simulink model "Tarea_4"  (R2013a)
settings: Solver=ode23s  StartTime=0.0  StopTime=10.0  RelTol=1e-3
libraries: simulink x6
settings Model: Creator=Miguel  LastModifiedBy=Miguel
settings DataIOCC: LimitDataPoints=off  MaxDataPoints=10000

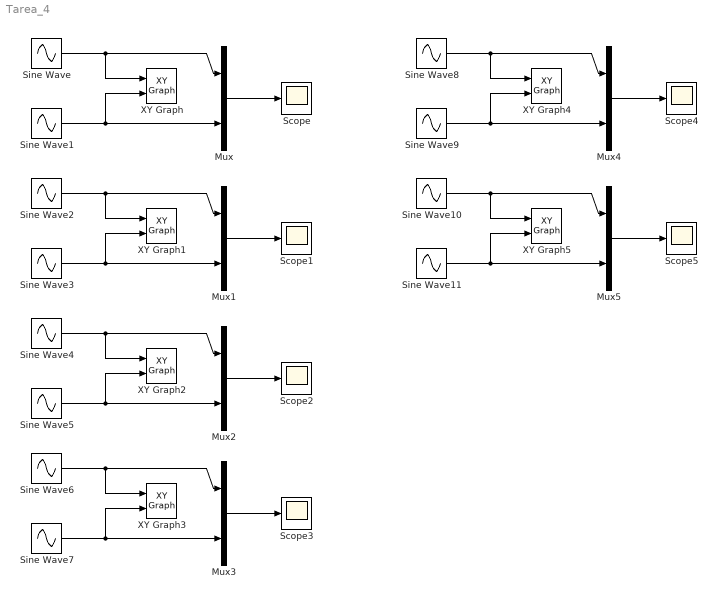
== system Tarea_4 ==
  Mux{,1..5} (6 alike) : Mux  Inputs=2
  Scope{,1..5} (6 alike) : Scope
      Scope settings: TickLabels=on  ShowLegends=on
      Scope1 settings: TickLabels=on  ShowLegends=on
      Scope2 settings: TickLabels=on  ShowLegends=on  SaveName=ScopeData2
      Scope3 settings: TickLabels=on  ShowLegends=on  SaveName=ScopeData3
      Scope4 settings: TickLabels=on  ShowLegends=on  SaveName=ScopeData4
      Scope5 settings: TickLabels=on  ShowLegends=on  SaveName=ScopeData5
  Sine Wave : Sin  Amplitude=2  SampleTime=0
  Sine Wave1 : Sin  Amplitude=2  Frequency=2  Phase=pi/4  SampleTime=0
  Sine Wave10 : Sin  Frequency=16  SampleTime=0
  Sine Wave11 : Sin  Frequency=9  Phase=pi/16  SampleTime=0
  Sine Wave2 : Sin  Amplitude=2  SampleTime=0
  Sine Wave3 : Sin  Amplitude=2  Frequency=2  Phase=pi/4  SampleTime=0
  Sine Wave4 : Sin  SampleTime=0
  Sine Wave5 : Sin  Frequency=4  Phase=pi/3  SampleTime=0
  Sine Wave6 : Sin  SampleTime=0
  Sine Wave7 : Sin  Phase=pi/2  SampleTime=0
  Sine Wave8 : Sin  Frequency=2  SampleTime=0
  Sine Wave9 : Sin  Frequency=3  SampleTime=0
  XY Graph : simulink/Sinks/XY Graph  xmin=-1  xmax=1  ymin=-1  ymax=1  st=-1
  XY Graph1 : simulink/Sinks/XY Graph  xmin=-3  xmax=3  ymin=-3  ymax=3  st=-1
  XY Graph2 : simulink/Sinks/XY Graph  xmin=-2  xmax=2  ymin=-2  ymax=2  st=-1
  XY Graph3 : simulink/Sinks/XY Graph  xmin=-1  xmax=1  ymin=-1  ymax=1  st=-1
  XY Graph4 : simulink/Sinks/XY Graph  xmin=-1  xmax=1  ymin=-1  ymax=1  st=-1
  XY Graph5 : simulink/Sinks/XY Graph  xmin=-2  xmax=2  ymin=-2  ymax=2  st=-1
  wires:
  Mux/1 -> Scope/1
  Sine Wave/1 -> Mux/1, XY Graph/1
  Sine Wave1/1 -> XY Graph/2, Mux/2
  Mux1/1 -> Scope1/1
  Sine Wave2/1 -> Mux1/1, XY Graph1/1
  Sine Wave3/1 -> XY Graph1/2, Mux1/2
  Mux2/1 -> Scope2/1
  Sine Wave4/1 -> Mux2/1, XY Graph2/1
  Sine Wave5/1 -> XY Graph2/2, Mux2/2
  Mux3/1 -> Scope3/1
  Sine Wave6/1 -> Mux3/1, XY Graph3/1
  Sine Wave7/1 -> XY Graph3/2, Mux3/2
  Mux4/1 -> Scope4/1
  Sine Wave8/1 -> Mux4/1, XY Graph4/1
  Sine Wave9/1 -> XY Graph4/2, Mux4/2
  Mux5/1 -> Scope5/1
  Sine Wave10/1 -> Mux5/1, XY Graph5/1
  Sine Wave11/1 -> XY Graph5/2, Mux5/2
